simulink model "Sistema_fisico_completo"  (R2023b)
settings: Solver=VariableStepAuto  StartTime=0.0  StopTime=10.0  RelTol=1e-3
settings Model: Creator=rodri  LastModifiedBy=Nahuel

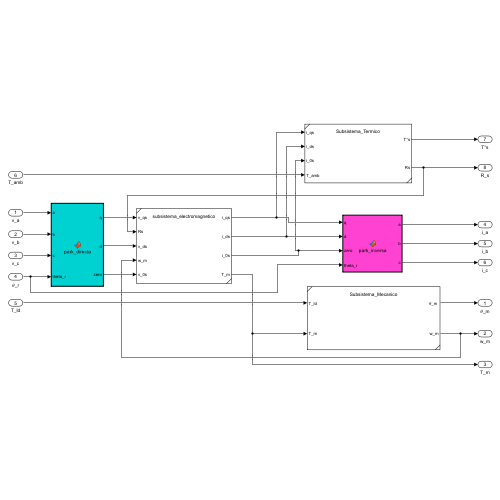
[thumbnail: Simulink's stored preview of the top-level diagram]
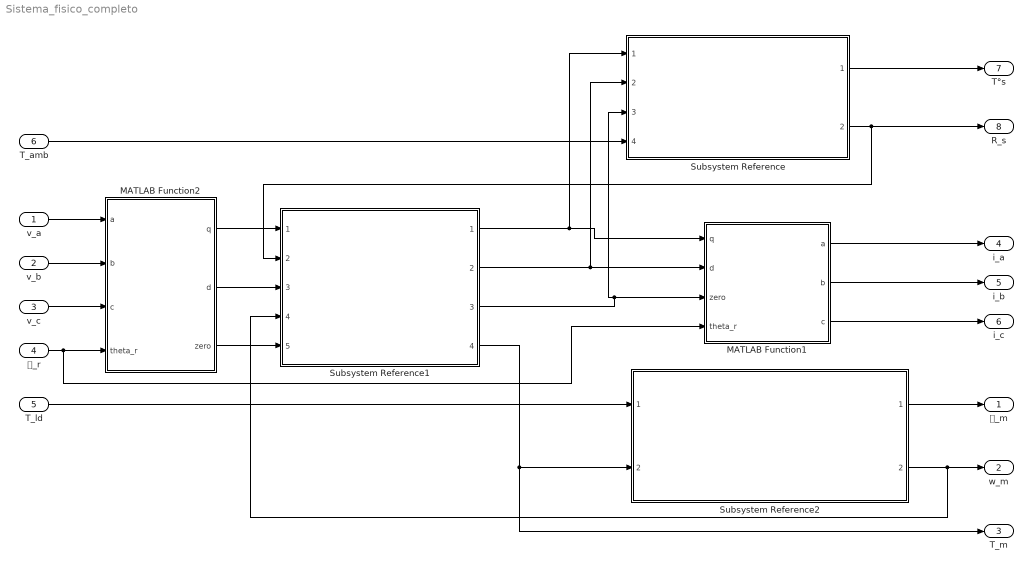
== system Sistema_fisico_completo ==
  v_a : Inport
  v_b : Inport  Port=2
  v_c : Inport  Port=3
  𝜃_r : Inport  Port=4
  T_ld : Inport  Port=5
  T_amb : Inport  Port=6
  MATLAB Function1 : MATLAB Function  TreatAsAtomicUnit=on
  MATLAB Function2 : MATLAB Function  TreatAsAtomicUnit=on
  Subsystem Reference : Subsystem  ReferencedSubsystem=Subsistema_Termico
  Subsystem Reference1 : Subsystem  ReferencedSubsystem=subsistema_electromagnetico
  Subsystem Reference2 : Subsystem  ReferencedSubsystem=Subsistema_Mecanico
  𝜃_m : Outport
  w_m : Outport  Port=2
  T_m : Outport  Port=3
  i_a : Outport  Port=4
  i_b : Outport  Port=5
  i_c : Outport  Port=6
  T°s : Outport  Port=7
  R_s : Outport  Port=8
  wires:
  v_b/1 -> MATLAB Function2/2(b)
  v_a/1 -> MATLAB Function2/1(a)
  v_c/1 -> MATLAB Function2/3(c)
  𝜃_r/1 -> MATLAB Function2/4(theta_r), MATLAB Function1/4(theta_r)
  MATLAB Function2/2(d) -> Subsystem Reference1/3
  MATLAB Function2/1(q) -> Subsystem Reference1/1
  MATLAB Function2/3(zero) -> Subsystem Reference1/5
  T_ld/1 -> Subsystem Reference2/1
  Subsystem Reference1/4 -> T_m/1, Subsystem Reference2/2
  Subsystem Reference1/1 -> MATLAB Function1/1(q), Subsystem Reference/1
  Subsystem Reference1/2 -> MATLAB Function1/2(d), Subsystem Reference/2
  Subsystem Reference1/3 -> MATLAB Function1/3(zero), Subsystem Reference/3
  T_amb/1 -> Subsystem Reference/4
  Subsystem Reference2/1 -> 𝜃_m/1
  Subsystem Reference2/2 -> w_m/1, Subsystem Reference1/4
  MATLAB Function1/1(a) -> i_a/1
  MATLAB Function1/3(c) -> i_c/1
  MATLAB Function1/2(b) -> i_b/1
  Subsystem Reference/2 -> Subsystem Reference1/2, R_s/1
  Subsystem Reference/1 -> T°s/1

== matlab function Sistema_fisico_completo/MATLAB Function1 ==
  data: q input; a output; d input; zero input; theta_r input; b output; c output
function [a, b, c] = park_inversa(q, d, zero, theta_r)
    % Transformación de Park Inversa
    % Entradas:
    %   d, q, z: Coordenadas en el marco rotatorio
    %   theta: Ángulo en radianes
    % Salidas:
    %   a, b, c: Valores trifásicos reconstruidos
    
    % Constantes
    alpha = 2 * pi / 3; % Desplazamiento angular entre fases
    
    % Cálculo de valores trifásicos
    a = q * cos(theta_r) + d * sin(theta_r) + zero;
    b = q * cos(theta_r - alpha) + d * sin(theta_r - alpha) + zero;
    c = q * cos(theta_r + alpha) + d * sin(theta_r + alpha) + zero;
end

== matlab function Sistema_fisico_completo/MATLAB Function2 ==
  data: q output; a input; d output; b input; c input; theta_r input; zero output
function [q, d, zero] = park_directa(a, b, c, theta_r)
    % Transformación de Park Directa
    % Entradas:
    %   a, b, c: Valores trifásicos
    %   theta: Ángulo en radianes
    % Salidas:
    %   d, q, z: Coordenadas en el marco rotatorio
    
    % Constantes
    alpha = 2 * pi / 3; % Desplazamiento angular entre fases
    k = 2 / 3; % Escala para invarianza
    
    % Cálculo de coordenadas d, q, z
    q = k * (a * cos(theta_r) + b * cos(theta_r - alpha) + c * cos(theta_r + alpha));
    d = k * (a * sin(theta_r) + b * sin(theta_r - alpha) + c * sin(theta_r + alpha));
    zero = k * (a * 1/2 + b * 1/2 + c * 1/2);
end
